simulink model "cw6_model_Relidzynski"  (R2017b)
settings: Solver=VariableStepAuto  StartTime=1  StopTime=200  RelTol=1e-3
undefined symbols (not defined in the file): a11, a12, a21, a22, b1
settings Model: Creator=Radek  LastModifiedBy=Radosław
settings DataIOCC: ReturnWorkspaceOutputs=on
settings DebuggingCC: UnconnectedInputMsg=none  UnconnectedOutputMsg=none  UnconnectedLineMsg=none  SFMachineParentedDataDiag=error
settings SFSimCC: SimUseLocalCustomCode=on
settings RTWCC: RTWUseLocalCustomCode=on

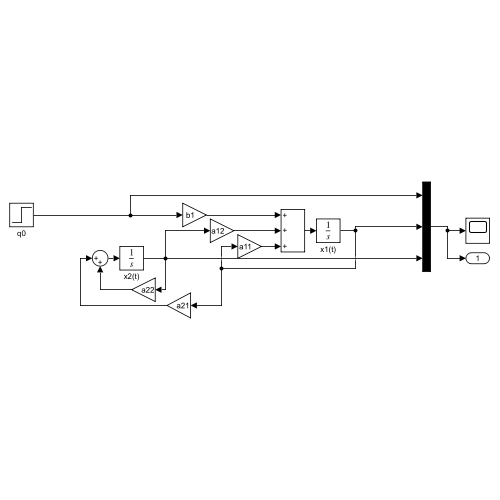
[thumbnail: Simulink's stored preview of the top-level diagram]
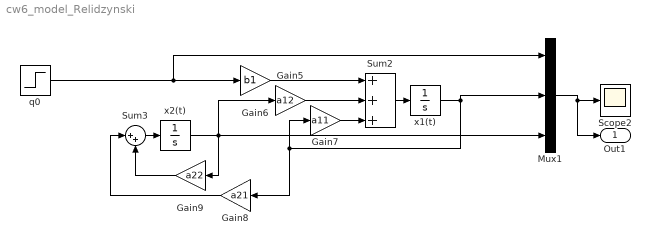
== system cw6_model_Relidzynski ==
  Gain5 : Gain  Gain=a12
  Gain6 : Gain  Gain=b1
  Gain7 : Gain  Gain=a11
  Gain8 : Gain  Gain=a21
  Gain9 : Gain  Gain=a22
  Mux1 : Mux  Inputs=3
  Scope2 : Scope
  Sum2 : Sum  Inputs=+++
  Sum3 : Sum  Inputs=|++
  q0 : Step  SampleTime=0
  x1(t) : Integrator
  x2(t) : Integrator
  Out1 : Outport
  wires:
  Gain7/1 -> Sum2/3
  Gain5/1 -> Sum2/2
  Sum3/1 -> x2(t)/1
  Sum2/1 -> x1(t)/1
  x1(t)/1 -> Gain8/1, Gain7/1, Mux1/2
  q0/1 -> Mux1/1, Gain6/1
  x2(t)/1 -> Mux1/3, Gain5/1, Gain9/1
  Gain8/1 -> Sum3/1
  Mux1/1 -> Out1/1, Scope2/1
  Gain9/1 -> Sum3/2
  Gain6/1 -> Sum2/1
